simulink library "ImageProcessing_cl"  (R2018b)
settings: Solver=VariableStepAuto  StartTime=0.0  StopTime=10.0  RelTol=1e-3
libraries: CalculateDistance_ul x1, dotFinder_ul x1, findDotCentroidPosition_ul x1, FindUnitVectorComponents_ul x1
settings Model: Creator=mcobb  LastModifiedBy=mcobb
settings DebuggingCC: LibraryContextMissingDiagnostic=none
settings SFSimCC: SimUseLocalCustomCode=off
settings RTWCC: RTWUseLocalCustomCode=off

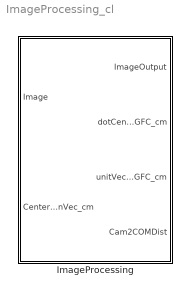
== system ImageProcessing_cl ==
  ImageProcessing : Subsystem  TreatAsAtomicUnit=on  mask{ROIPositionHoldEnable=on, ROIPositionHoldCoordinates=[500 500], ROIDimVec_px=[30 90], ROIHalfDimVec_px=[15 45], ROISplitDims_px=[1 15 ; 1 90 ; 16 14 ; 1 90], DotOrientation=Vertical, OverlayOutput=on, ImageDimensions=[765 998], CrosshairPixelWidth_px=1, cameraSelection=Side, camPositionVec_cm=[20 -50 50], camFOVVec_deg=[30 30]}
      mask prompts: ROIPositionHoldEnable "Hold Position Enable"; ROIPositionHoldCoordinates "Hold Position Coordinates  [rows cols]  (pixels)"; ROIDimVec_px "Dimensions [rows cols]  (pixels)"; ROIHalfDimVec_px "Half Dims  [rows cols]  (pixels)"; ROISplitDims_px "Split Dims [rows cols]  (pixels)"; DotOrientation "Dot Orientation"; OverlayOutput "Draw Output Overlay"; ImageDimensions "Image Dimensions [rows cols] pixels"; CrosshairPixelWidth_px "Crosshair Width (pixels)"; cameraSelection "Camera Selection"; camPositionVec_cm "Camera Position Vector [x y z] cm"; camFOVVec_deg "Camera Field of View [horiz vert] deg"
      mask help:
      | This block does all the image processing necessary to find the dots, then find the relevant components of the unit vector in question.
      |
      | Written 10/17/2018 - MC
      mask init:
      | imageProcessingInit
      mask TypeOptions DotOrientation: Horizontal | Vertical
      mask TypeOptions cameraSelection: sortComponents/cameraSelection
      mask DialogControl ParameterGroupVar Prompt: Region Of Interest (ROI) Parameters
      mask DialogControl Container3 Prompt: Other Parameters

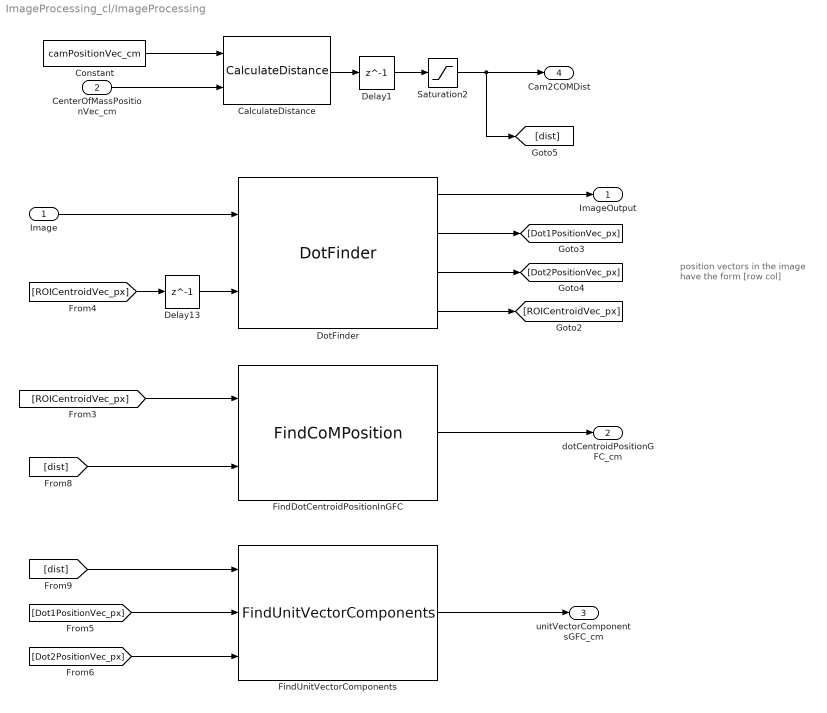
== system ImageProcessing_cl/ImageProcessing ==
  note: position vectors in the image
      | have the form [row col]
  "Image " : Inport
  "CenterOfMassPositionVec_cm " : Inport  Port=2
  CalculateDistance : CalculateDistance_ul/CalculateDistance  SystemSampleTime=-1
  Constant : Constant  Value=camPositionVec_cm
  Delay1 : Delay  DelayLength=1  InitialCondition=1
  Delay13 : Delay  DelayLength=1  InitialCondition=1460
  DotFinder : dotFinder_ul/DotFinder  ROIPositionHoldEnable=on  ROIPositionHoldCoordinates=ROIPositionHoldCoordinates  ROIDimVec_px=ROIDimVec_px  ROIHalfDimVec_px=[15 45]  ROISplitDims_px=[1 15 ; 1 90 ; 16 14 ; 1 90]  DotOrientation=Vertical  OverlayOutput=on  ImageDimensions=ImageDimensions  CrosshairPixelWidth_px=CrosshairPixelWidth_px
  FindDotCentroidPositionInGFC : findDotCentroidPosition_ul/FindCoMPosition  camPositionVec_cm=camPositionVec_cm  cameraViewAngleVec_deg=camFOVVec_deg  cam2GroundRotationMatrix=cam2GroundRotationMatrix  imageDimensions_px=ImageDimensions
  FindUnitVectorComponents : FindUnitVectorComponents_ul/FindUnitVectorComponents  cameraViewAngleVec_deg=camFOVVec_deg  cam2GroundRotationMatrix=cam2GroundRotationMatrix  imageDimensions=imageDimensions
  Saturation2 : Saturate  UpperLimit=200  LowerLimit=1
  ImageOutput : Outport
  dotCentroidPositionGFC_cm : Outport  Port=2
  unitVectorComponentsGFC_cm : Outport  Port=3
  Cam2COMDist : Outport  Port=4
  wires:
  FindDotCentroidPositionInGFC/1 -> dotCentroidPositionGFC_cm/1
  "Image "/1 -> DotFinder/1
  DotFinder/1 -> ImageOutput/1
  CalculateDistance/1 -> Delay1/1
  "CenterOfMassPositionVec_cm "/1 -> CalculateDistance/2
  Delay1/1 -> Saturation2/1
  Delay13/1 -> DotFinder/2
  DotFinder/4 -> [ROICentroidVec_px]
  [ROICentroidVec_px] -> Delay13/1
  [Dot1PositionVec_px] -> FindUnitVectorComponents/2
  [Dot2PositionVec_px] -> FindUnitVectorComponents/3
  DotFinder/2 -> [Dot1PositionVec_px]
  DotFinder/3 -> [Dot2PositionVec_px]
  Saturation2/1 -> Cam2COMDist/1, [dist]
  [dist] -> FindUnitVectorComponents/1
  Constant/1 -> CalculateDistance/1
  [dist] -> FindDotCentroidPositionInGFC/2
  [ROICentroidVec_px] -> FindDotCentroidPositionInGFC/1
  FindUnitVectorComponents/1 -> unitVectorComponentsGFC_cm/1
